simulink model "extra_task_PID"  (R2021b)
settings: Solver=FixedStepAuto  StartTime=0.0  StopTime=20  FixedStep=0.001  RelTol=1e-3
values from neighbouring files (symbols this model uses):
  hd = 1.2    [mass_1dof.m]
  hi = 0    [mass_1dof.m]
  hp = 0    [mass_1dof.m]
  kp = 6.32    [mass_1dof.m]    (also in mass_2dof.m)
  mp = 0.16    [mass_1dof.m]    (also in mass_2dof.m)
settings Model: Creator=rivaa  LastModifiedBy=rivaa

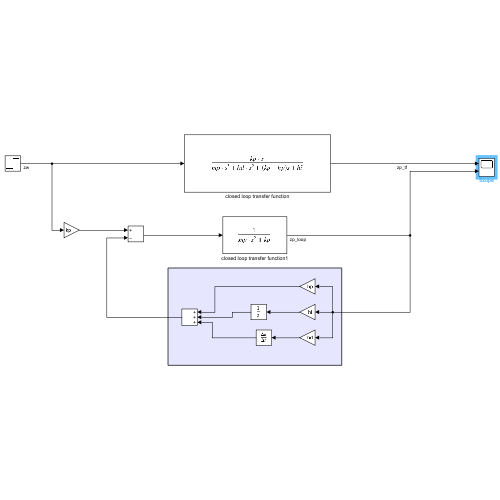
[thumbnail: Simulink's stored preview of the top-level diagram]
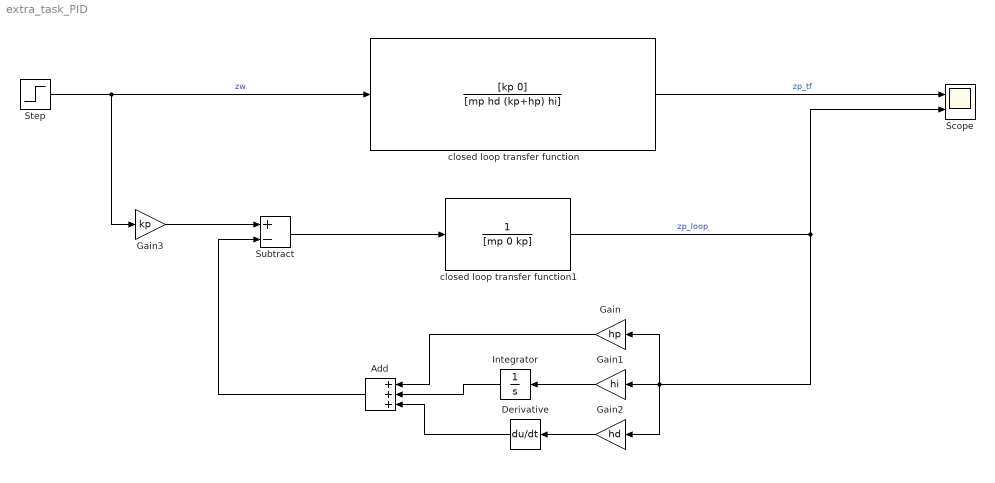
== system extra_task_PID ==
  Add : Sum  Inputs=+++
  Derivative : Derivative
  Gain : Gain  Gain=hp
  Gain1 : Gain  Gain=hi
  Gain2 : Gain  Gain=hd
  Gain3 : Gain  Gain=kp
  Integrator : Integrator
  Scope : Scope  NumInputPorts=2
  Step : Step  Time=0  SampleTime=0
  Subtract : Sum  Inputs=+-
  closed loop transfer function : TransferFcn  Numerator=[kp 0]  Denominator=[mp hd (kp+hp) hi]
  closed loop transfer function1 : TransferFcn  Numerator=1  Denominator=[mp 0 kp]
  wires:
  Step/1 -> closed loop transfer function/1, Gain3/1  "zw"
  Gain1/1 -> Integrator/1
  Gain2/1 -> Derivative/1
  Gain/1 -> Add/1
  Integrator/1 -> Add/2
  Derivative/1 -> Add/3
  closed loop transfer function/1 -> Scope/1  "zp_tf"
  Gain3/1 -> Subtract/1
  Subtract/1 -> closed loop transfer function1/1
  closed loop transfer function1/1 -> Scope/2, Gain2/1, Gain/1, Gain1/1  "zp_loop"
  Add/1 -> Subtract/2
